simulink model "test_quaternions"  (R2023b)
settings: Solver=FixedStepAuto  StartTime=0.0  StopTime=inf  FixedStep=0.005  RelTol=1e-3
libraries: sharedtransform x9, simulink_extras x8, shared6dof x1, aerolibutil x1, sharedutil x1
settings Model: Creator=frank  LastModifiedBy=frank

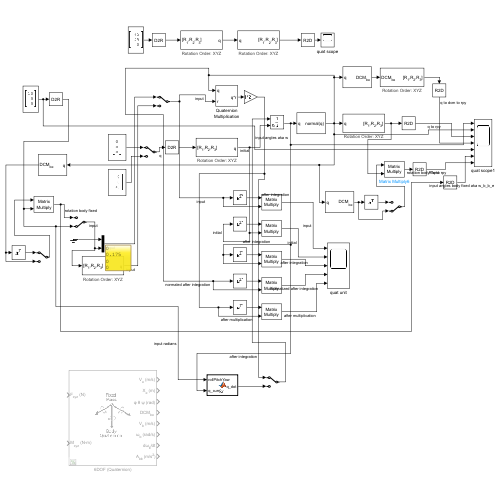
[thumbnail: Simulink's stored preview of the top-level diagram]
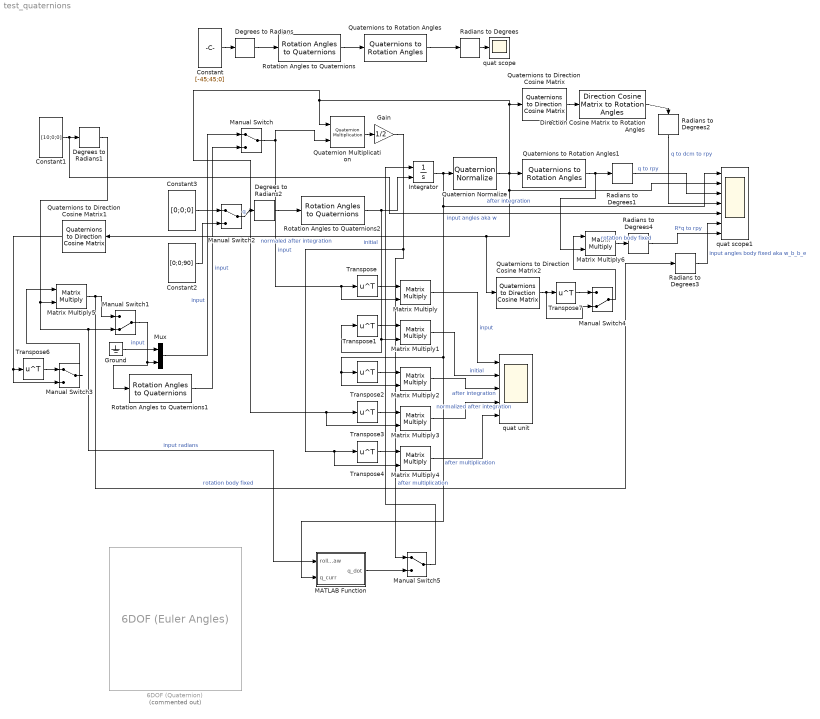
== system test_quaternions ==
  6DOF (Quaternion) : shared6dof/6DOF (Euler Angles)  Commented=on  units=Metric (MKS)  mtype=Fixed  rep=Quaternion  xme_0=[0 0 0]  Vm_0=[0 0 0]  eul_0=[0 0 0]  pm_0=[0 0 0]  mass_0=1.0  mass_e=0.5  mass_f=2.0  inertia=eye(3)  inertia_e=eye(3)  inertia_f=2*eye(3)  k_quat=1.0  vre_flag=on  abi_flag=off  aMode=0  xme_statename=''  Vm_statename=''  eul_statename=''  quat_statename=''  pm_statename=''  mass_statename=''
      settings: LibrarySourceBlock=aerolib6dof2/6DOF (Quaternion)
  Constant : Constant  Value=[-45;45;0]  VectorParams1D=off
  Constant1 : Constant  Value=[10;0;0]  VectorParams1D=off
  Constant2 : Constant  Value=[0;0;90]  VectorParams1D=off
  Constant3 : Constant  Value=[0;0;0]  VectorParams1D=off
  Degrees to Radians : simulink_extras/Transformations/Degrees to Radians
  Degrees to Radians1 : simulink_extras/Transformations/Degrees to Radians
  Degrees to Radians2 : simulink_extras/Transformations/Degrees to Radians
  Direction Cosine Matrix to Rotation Angles : sharedtransform/Direction Cosine Matrix to Rotation Angles  rotationOrder=XYZ  aMode=aMode  action=None  tolerance=eps(2)
      settings: LibrarySourceBlock=|
      | aerolibtransform2/Direction Cosine Matrix
      | to Rotation Angles
  Gain : Gain  Gain=1/2
  Ground : Ground
  Integrator : Integrator  InitialConditionSource=external
  MATLAB Function : MATLAB Function  TreatAsAtomicUnit=on
  Manual Switch{,2..3,5} (4 alike) : ManualSwitch
  Manual Switch1 : ManualSwitch  CurrentSetting=0
  Manual Switch4 : ManualSwitch  CurrentSetting=0
  Matrix Multiply{,1..6} (7 alike) : Product  Multiplication=Matrix(*)
  Mux : Mux  Inputs=2
  Quaternion Multiplication : aerolibutil/Quaternion Multiplication
  Quaternion Normalize : sharedutil/Quaternion Normalize  aMode=aMode
  Quaternions to Direction Cosine Matrix : sharedtransform/Quaternions to  Direction Cosine Matrix  aMode=aMode
      settings: LibrarySourceBlock=|
      | aerolibtransform2/Quaternions to
      | Direction Cosine Matrix
  Quaternions to Direction Cosine Matrix1 : sharedtransform/Quaternions to  Direction Cosine Matrix  aMode=aMode
      settings: LibrarySourceBlock=|
      | aerolibtransform2/Quaternions to
      | Direction Cosine Matrix
  Quaternions to Direction Cosine Matrix2 : sharedtransform/Quaternions to  Direction Cosine Matrix  aMode=aMode
      settings: LibrarySourceBlock=|
      | aerolibtransform2/Quaternions to
      | Direction Cosine Matrix
  Quaternions to Rotation Angles : sharedtransform/Quaternions to Rotation Angles  rotationOrder=XYZ  aMode=aMode
  Quaternions to Rotation Angles1 : sharedtransform/Quaternions to Rotation Angles  rotationOrder=XYZ  aMode=aMode
  Radians to Degrees{,1..4} (5 alike) : simulink_extras/Transformations/Radians to Degrees
  Rotation Angles to Quaternions : sharedtransform/Rotation Angles to Quaternions  rotationOrder=XYZ  aMode=aMode
  Rotation Angles to Quaternions1 : sharedtransform/Rotation Angles to Quaternions  rotationOrder=XYZ  aMode=aMode
  Rotation Angles to Quaternions2 : sharedtransform/Rotation Angles to Quaternions  rotationOrder=XYZ  aMode=aMode
  Transpose{,1..4,6..7} (7 alike) : Math  Operator=transpose
  quat scope : Scope
  quat scope1 : Scope  NumInputPorts=7
  quat unit : Scope  NumInputPorts=5
  wires:
  Constant/1 -> Degrees to Radians/1
  Rotation Angles to Quaternions/1 -> Quaternions to Rotation Angles/1
  Quaternions to Rotation Angles/1 -> Radians to Degrees/1
  Degrees to Radians/1 -> Rotation Angles to Quaternions/1
  Radians to Degrees/1 -> quat scope/1
  Degrees to Radians1/1 -> Manual Switch1/2, MATLAB Function/1(rollPitchYaw), Matrix Multiply5/2  "input radians"
  Constant1/1 -> quat scope1/5, Degrees to Radians1/1  "input angles aka w"
  Manual Switch/1 -> Matrix Multiply/2, Transpose/1, Quaternion Multiplication/2  "input"
  Radians to Degrees1/1 -> quat scope1/3  "q to rpy"
  Constant2/1 -> Manual Switch2/2
  Manual Switch2/1 -> Degrees to Radians2/1  "q"
  Constant3/1 -> Manual Switch2/1
  Degrees to Radians2/1 -> Rotation Angles to Quaternions2/1
  Rotation Angles to Quaternions2/1 -> Transpose1/1, Matrix Multiply1/2, Integrator/2  "initial"
  Integrator/1 -> MATLAB Function/2(q_curr), Matrix Multiply2/2, Transpose2/1, quat scope1/1, Quaternion Normalize/1  "after integration"
  Quaternions to Rotation Angles1/1 -> Matrix Multiply6/2, Radians to Degrees1/1
  Quaternion Normalize/1 -> Quaternions to Direction Cosine Matrix2/1, Quaternions to Direction Cosine Matrix1/1, quat scope1/2, Quaternion Multiplication/1, Matrix Multiply3/2, Transpose3/1, Quaternions to Direction Cosine Matrix/1, Quaternions to Rotation Angles1/1  "normaled after integration"
  Quaternion Multiplication/1 -> Gain/1
  Gain/1 -> Manual Switch5/1, Matrix Multiply4/2, Transpose4/1  "after multiplication"
  Transpose/1 -> Matrix Multiply/1
  Transpose1/1 -> Matrix Multiply1/1
  Transpose2/1 -> Matrix Multiply2/1
  Transpose3/1 -> Matrix Multiply3/1
  Transpose4/1 -> Matrix Multiply4/1
  Matrix Multiply/1 -> quat unit/1  "input"
  Matrix Multiply1/1 -> quat unit/2  "initial"
  Matrix Multiply2/1 -> quat unit/3  "after integration"
  Matrix Multiply3/1 -> quat unit/4  "normalized after integration"
  Matrix Multiply4/1 -> quat unit/5  "after multiplication"
  Ground/1 -> Mux/1
  Quaternions to Direction Cosine Matrix/1 -> Direction Cosine Matrix to Rotation Angles/1
  Direction Cosine Matrix to Rotation Angles/1 -> Radians to Degrees2/1
  Radians to Degrees2/1 -> quat scope1/4  "q to dcm to rpy"
  Mux/1 -> Manual Switch/1  "input"
  Rotation Angles to Quaternions1/1 -> Manual Switch/2  "input"
  Quaternions to Direction Cosine Matrix1/1 -> Manual Switch3/2, Transpose6/1
  Matrix Multiply5/1 -> Radians to Degrees3/1, Manual Switch1/1  "rotation body fixed"
  Manual Switch1/1 -> Rotation Angles to Quaternions1/1, Mux/2  "input"
  Radians to Degrees3/1 -> quat scope1/6  "input angles body fixed aka w_b_b_e"
  Matrix Multiply6/1 -> Radians to Degrees4/1  "rotation body fixed"
  Radians to Degrees4/1 -> quat scope1/7  "R*q to rpy"
  Manual Switch4/1 -> Matrix Multiply6/1
  Transpose6/1 -> Manual Switch3/1
  Manual Switch3/1 -> Matrix Multiply5/1
  Quaternions to Direction Cosine Matrix2/1 -> Manual Switch4/2, Transpose7/1
  Transpose7/1 -> Manual Switch4/1
  MATLAB Function/1(q_dot) -> Manual Switch5/2
  Manual Switch5/1 -> Integrator/1

== matlab function test_quaternions/MATLAB Function ==
  data: rollPitchYaw input; q_dot output; q_curr input
function q_dot = fcn(rollPitchYaw,q_curr)

p = rollPitchYaw(1);%roll
q = rollPitchYaw(2);%pitch
r = rollPitchYaw(3);%yaw

rpy_matrix = [
    0,  -p, -q, -r
    p,  0,  r,  -q
    q,  -r, 0,  p
    r,  q,  -p, 0
    ];

K = 1;%normalization gait
epsilon = 1 - (q_curr(1)^2 + q_curr(2)^2 + q_curr(3)^2+q_curr(4)^2);

q_dot = (1/2)*rpy_matrix*q_curr + K*epsilon*q_curr;
